simulink model "Control_Logic_a"  (R2018b)
settings: Solver=VariableStepAuto  StartTime=Start_time  StopTime=Stop_time  RelTol=1e-3
values from neighbouring files (symbols this model uses):
  Aset_N1 = 2    [Parameter_control.m]
  Aset_N10 = -10    [Parameter_control.m]
  Aset_N11 = 10    [Parameter_control.m]
  Aset_N12 = 20    [Parameter_control.m]
  Aset_N13 = 20    [Parameter_control.m]
  Aset_N2 = 30    [Parameter_control.m]
  Aset_N3 = 3    [Parameter_control.m]
  Aset_N4 = 5    [Parameter_control.m]
  Aset_N5 = 1    [Parameter_control.m]
  Aset_N6 = 0    [Parameter_control.m]
  Aset_N7 = 0.01    [Parameter_control.m]
  Aset_N8 = 2    [Parameter_control.m]
  Aset_N9 = 0.1    [Parameter_control.m]
  Dset_N1 = 1    [Parameter_control.m]
  Dset_N2 = 1    [Parameter_control.m]
  Ini_time = Start_time    (= 0)    [main.m]
  Sample_time = 0.1    [main.m]    (also in manual_env_for_test_slx.m; test_tool_initialize.m)
undefined symbols (not defined in the file or in its folder): DiscIntNeverNeededParam
(part 1 of 2)
settings Model: Creator=M156732  LastModifiedBy=M156732
settings ModelReferenceCC: ModelReferenceNumInstancesAllowed=Single

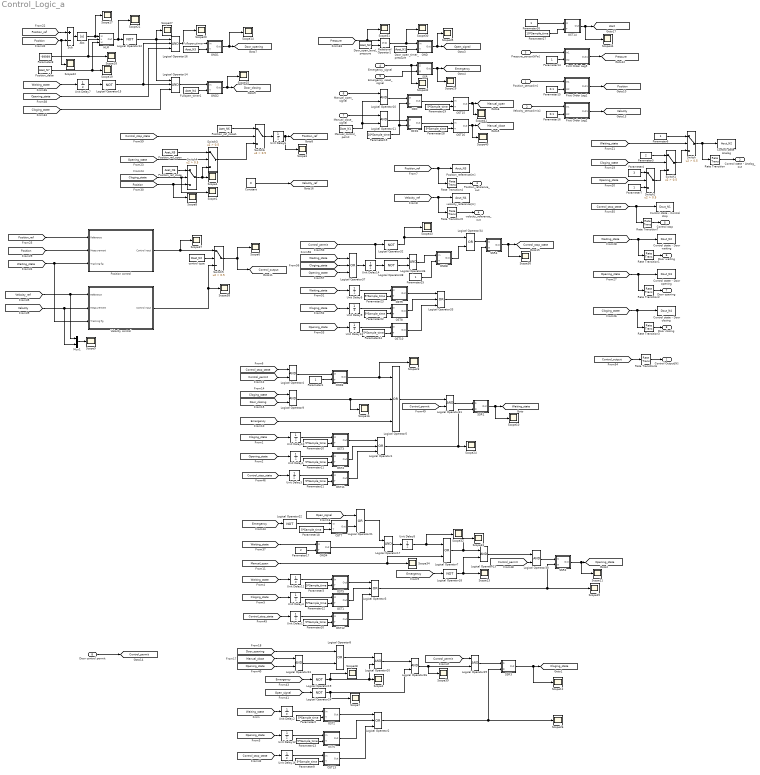
== system Control_Logic_a ==
  Position_sensor[m] : Inport  OutDataTypeStr=double  Unit=mm  SampleTime=Sample_time
  Velocity_sensor[m/s] : Inport  Port=2  OutDataTypeStr=double  Unit=mm  SampleTime=Sample_time
  Pressure_sensor[kPa] : Inport  Port=3  OutDataTypeStr=double  Unit=kPa  SampleTime=Sample_time
  Emergency_signal : Inport  Port=4  OutDataTypeStr=boolean  SampleTime=Sample_time
  Emergency_reset_signal : Inport  Port=5  OutDataTypeStr=boolean  SampleTime=Sample_time
  Manual_open_signal : Inport  Port=6  OutDataTypeStr=boolean  SampleTime=Sample_time
  Manual_close_signal : Inport  Port=7  OutDataTypeStr=boolean  SampleTime=Sample_time
  Door control permit : Inport  Port=8  OutDataTypeStr=boolean  SampleTime=Sample_time
  Abs : Abs
  Constant : Constant  Value=0
  Control state - Analog : ToWorkspace  VariableName=Aout_N2  SampleTime=Sample_time
  Control state - Control stop : ToWorkspace  VariableName=Dout_N1  SampleTime=Sample_time
  Control state - Door closing : ToWorkspace  VariableName=Dout_N4  SampleTime=Sample_time
  Control state - Door opening : ToWorkspace  VariableName=Dout_N3  SampleTime=Sample_time
  Control state - Door waiting : ToWorkspace  VariableName=Dout_N2  SampleTime=Sample_time
  Door_open_level_pressure : Constant  Value=Aset_N2  OutDataTypeStr=double  SampleTime=Sample_time
  Door_open_timer_pressure : Constant  Value=Aset_N1  OutDataTypeStr=double  SampleTime=Sample_time
  First Order Lag1 : Subsystem
  First Order Lag2 : Subsystem
  First Order Lag5 : Subsystem
  Fullopen_timer : Constant  Value=Aset_N3  OutDataTypeStr=double  SampleTime=Sample_time
  Fullopen_timer1 : Constant  Value=Aset_N4  OutDataTypeStr=double  SampleTime=Sample_time
  HLM : Subsystem
  Logical Operator{1..3,5,33,37} (6 alike) : Logic  Operator=OR  Inputs=3  AllPortsSameDT=off  OutDataTypeStr=boolean
  Logical Operator{4,9..11,13,17,20,23,26,29..31,36} (13 alike) : Logic  AllPortsSameDT=off  OutDataTypeStr=boolean
  Logical Operator{12,15,18..19,22,24,32,38} (8 alike) : Logic  Operator=NOT  AllPortsSameDT=off  OutDataTypeStr=boolean
  Logical Operator14 : Logic  Inputs=3  AllPortsSameDT=off  OutDataTypeStr=boolean
  Logical Operator16 : Logic  Inputs=3  AllPortsSameDT=off  OutDataTypeStr=boolean
  Logical Operator{7..8,21,34} (4 alike) : Logic  Operator=OR  AllPortsSameDT=off  OutDataTypeStr=boolean
  Manual_control_pemit : Constant  Value=Dset_N1  OutDataTypeStr=double  SampleTime=Sample_time
  Mux1 : Mux  Inputs=2
  OFD : Subsystem
  OFD1 : Subsystem
  OND : Subsystem
  OND1 : Subsystem
  OND2 : Subsystem
  OND3 : Subsystem
  OND4 : Subsystem
  OND8 : Subsystem
  OST1 : Subsystem
  OST10 : Subsystem
  OST11 : Subsystem
  OST12 : Subsystem
  OST13 : Subsystem
  OST14 : Subsystem
  OST15 : Subsystem
  OST16 : Subsystem
  OST2 : Subsystem
  OST3 : Subsystem
  OST4 : Subsystem
  OST5 : Subsystem
  OST6 : Subsystem
  OST7 : Subsystem
  OST8 : Subsystem
  OST9 : Subsystem
  Parameter{1,6..7,25} (4 alike) : Constant  OutDataTypeStr=int32  SampleTime=Sample_time
  Parameter{2..3,9..13,18,20..24,28..29} (15 alike) : Constant  Value=5*Sample_time  OutDataTypeStr=double  SampleTime=Sample_time
  Parameter14 : Constant  OutDataTypeStr=double  SampleTime=Sample_time
  Parameter15 : Constant  Value=0.1  OutDataTypeStr=double  SampleTime=Sample_time
  Parameter16 : Constant  Value=0.1  OutDataTypeStr=double  SampleTime=Sample_time
  Parameter17 : Constant  Value=2  OutDataTypeStr=int32  SampleTime=Sample_time
  Parameter19 : Constant  Value=10*Sample_time  OutDataTypeStr=double  SampleTime=Sample_time
  Parameter26 : Constant  OutDataTypeStr=boolean  SampleTime=Sample_time
  Parameter27 : Constant  Value=10*Sample_time  OutDataTypeStr=double  SampleTime=Sample_time
  Parameter4 : Constant  Value=3  OutDataTypeStr=int32  SampleTime=Sample_time
  Parameter5 : Constant  Value=2  OutDataTypeStr=int32  SampleTime=Sample_time
  Parameter8 : Constant  Value=-99999  OutDataTypeStr=double  SampleTime=Sample_time
  Position control : Subsystem
  Position_delta : Constant  Value=Aset_N7  OutDataTypeStr=double  SampleTime=Sample_time
  Position_ref_close : Constant  Value=Aset_N6  OutDataTypeStr=double  SampleTime=Sample_time
  Position_ref_close1 : Constant  Value=Aset_N6  OutDataTypeStr=double  SampleTime=Sample_time
  Position_ref_open : Constant  Value=Aset_N5  OutDataTypeStr=double  SampleTime=Sample_time
  Position_reference[m] : ToWorkspace  VariableName=Aout_N3  SampleTime=Sample_time
  Rate Transition{,1..7} (8 alike) : RateTransition  OutPortSampleTime=Sample_time
  Relational Operator1 : RelationalOperator  OutDataTypeStr=boolean  RndMeth=Nearest
  SSR : Subsystem
  SSR1 : Subsystem
  SSR2 : Subsystem
  SSR3 : Subsystem
  SSR4 : Subsystem
  Scope{1..4,6..44} (43 alike) : Scope
  Sub : Sum  Inputs=+-  OutDataTypeStr=double
  Switch : Switch  Criteria=u2 > Threshold  Threshold=0.5  OutDataTypeStr=int32
  Switch1 : Switch  Criteria=u2 > Threshold  Threshold=0.5  OutDataTypeStr=int32
  Switch2 : Switch  Criteria=u2 > Threshold  Threshold=0.5  OutDataTypeStr=int32
  Switch{3..6} (4 alike) : Switch  Criteria=u2 > Threshold  Threshold=0.5  OutDataTypeStr=double
  Unit Delay{1..13,15..16} (15 alike) : UnitDelay  SampleTime=Sample_time
  Unit Delay14 : UnitDelay  InitialCondition=1  SampleTime=Sample_time
  Velocity control : Subsystem
  control type : Constant  Value=Dset_N2  OutDataTypeStr=double  SampleTime=Sample_time
  velocity_reference[m] : ToWorkspace  VariableName=Aout_N4  SampleTime=Sample_time
  Control Output[N] : Outport  OutDataTypeStr=double  Unit=N  SampleTime=Sample_time  LockScale=on
  Control state - Analog_out : Outport  Port=2  SampleTime=Sample_time
  Position_reference_out : Outport  Port=3  SampleTime=Sample_time
  velocity_reference_out : Outport  Port=4  SampleTime=Sample_time
  Control stop : Outport  Port=5  SampleTime=Sample_time
  Door waiting : Outport  Port=6  SampleTime=Sample_time
  Door opening : Outport  Port=7  SampleTime=Sample_time
  Door closing : Outport  Port=8  SampleTime=Sample_time
  tag scope: Cloging_state=global, Control_output=global, Control_permit=global, Control_stop_state=global, Door_closing=global, Door_opening=global, Emergency=global, Manual_close=global, Manual_open=global, Open_signal=global, Opening_state=global, Position=global, Position_ref=global, Pressure=global, Velocity=global, Velocity_ref=global, Waiting_state=global, start=global
  wires:
  SSR1/1(Out) -> Scope10/1, [Waiting_state]
  SSR3/1(Out) -> Scope12/1, [Cloging_state]
  SSR2/1(Out) -> Scope11/1, [Opening_state]
  Logical Operator9/1 -> Scope16/1, Logical Operator5/2
  [Emergency] -> Logical Operator5/3
  [Door_closing] -> Logical Operator9/2
  [Cloging_state] -> Logical Operator9/1
  [Manual_open] -> Scope34/1, Logical Operator7/2
  Logical Operator7/1 -> Logical Operator13/1, Scope33/1
  [Door_opening] -> Logical Operator8/1
  Door_open_timer_pressure/1 -> OND/2(T)
  Door_open_level_pressure/1 -> Relational Operator1/2
  Relational Operator1/1 -> Scope30/1, OND/1(In)
  OND/1(Out) -> Scope35/1, [Open_signal]
  SSR/1(Out) -> Scope29/1, [Emergency]
  Emergency_reset_signal/1 -> SSR/2(R)
  Switch1/1 -> Switch/3
  Switch2/1 -> Switch1/3
  Parameter4/1 -> Switch2/1
  Parameter5/1 -> Switch1/1
  Parameter6/1 -> Switch/1
  Parameter7/1 -> Switch2/3
  Switch/1 -> Rate Transition/1, Control state - Analog/1
  Manual_control_pemit/1 -> Logical Operator10/2, Logical Operator11/2
  [Position_ref] -> Sub/1
  Sub/1 -> Abs/1
  Position_delta/1 -> Scope19/1, HLM/3(H)
  Parameter8/1 -> Scope18/1, HLM/2(L)
  HLM/1(Out) -> Scope21/1, Logical Operator12/1
  Fullopen_timer/1 -> OND1/2(T)
  [Opening_state] -> Switch3/2
  Switch4/1 -> Scope4/1, Switch3/3
  [Cloging_state] -> Scope1/1, Switch4/2
  Position_ref_open/1 -> Switch3/1
  Position_ref_close/1 -> Switch4/1
  [Position] -> Scope8/1, Switch4/3
  Fullopen_timer1/1 -> OND2/2(T)
  [Waiting_state] -> Rate Transition1/1, Control state - Door waiting/1
  [Opening_state] -> Rate Transition2/1, Control state - Door opening/1
  [Cloging_state] -> Rate Transition3/1, Control state - Door closing/1
  [Position] -> Scope22/1, Sub/2
  Unit Delay6/1 -> Scope3/1, [Position_ref]
  [Pressure] -> Scope31/1, Relational Operator1/1
  Parameter1/1 -> OND3/2(T)
  Logical Operator4/1 -> OND3/1(In)
  OND3/1(Out) -> Scope23/1, Logical Operator5/1
  Abs/1 -> Scope17/1, HLM/1(In)
  OND1/1(Out) -> Scope14/1, [Door_opening]
  OND2/1(Out) -> Scope15/1, [Door_closing]
  [Waiting_state] -> Unit Delay7/1
  Logical Operator12/1 -> Logical Operator16/1, Scope27/1, Logical Operator14/1
  Logical Operator16/1 -> OND1/1(In), Scope20/1
  Logical Operator15/1 -> Logical Operator14/2, Logical Operator16/2
  Unit Delay7/1 -> Logical Operator15/1
  Logical Operator1/1 -> SSR1/2(R), Scope24/1
  Logical Operator17/1 -> Unit Delay8/1
  Unit Delay8/1 -> Scope32/1, Logical Operator7/1
  [Opening_state] -> Logical Operator16/3
  [Cloging_state] -> Logical Operator14/3
  Logical Operator14/1 -> OND2/1(In)
  [Opening_state] -> Unit Delay1/1
  [Cloging_state] -> Unit Delay10/1
  Parameter10/1 -> OST3/2(T)
  OST3/1(Out) -> Logical Operator1/1
  Unit Delay10/1 -> OST3/1(In)
  Unit Delay1/1 -> OST4/1(In)
  Parameter11/1 -> OST4/2(T)
  OST4/1(Out) -> Logical Operator1/2
  Parameter12/1 -> OST1/2(T)
  Logical Operator3/1 -> SSR2/2(R), Scope25/1
  OST1/1(Out) -> Logical Operator3/2
  Parameter3/1 -> OST5/2(T)
  [Waiting_state] -> Unit Delay11/1
  OST5/1(Out) -> Logical Operator3/1
  Unit Delay11/1 -> OST5/1(In)
  [Cloging_state] -> Unit Delay4/1
  Unit Delay4/1 -> OST1/1(In)
  [Waiting_state] -> Unit Delay2/1
  Parameter2/1 -> OST2/2(T)
  Logical Operator2/1 -> Scope26/1, SSR3/2(R)
  OST2/1(Out) -> Logical Operator2/1
  Parameter13/1 -> OST6/2(T)
  [Opening_state] -> Unit Delay12/1
  OST6/1(Out) -> Logical Operator2/2
  Unit Delay2/1 -> OST2/1(In)
  Unit Delay12/1 -> OST6/1(In)
  [Position_ref] -> Position control/1(Reference)
  [Position] -> Position control/2(Measurement)
  [Waiting_state] -> Velocity control/3(Tracking flg), Position control/3(Tracking flg)
  Position control/1(Control input) -> Scope37/1, Switch5/1
  Switch5/1 -> Scope6/1, [Control_output]
  Velocity control/1(Control input) -> Scope38/1, Switch5/3
  control type/1 -> Switch5/2
  [Velocity] -> Velocity control/2(Measurement), Mux1/2
  [Velocity_ref] -> Velocity control/1(Reference), Mux1/1
  Mux1/1 -> Scope9/1
  Pressure_sensor[kPa]/1 -> First Order Lag5/1(In1)
  First Order Lag5/1(Out1) -> [Pressure]
  First Order Lag1/1(Out1) -> [Position]
  Position_sensor[m]/1 -> First Order Lag1/1(In1)
  First Order Lag2/1(Out1) -> [Velocity]
  Velocity_sensor[m/s]/1 -> First Order Lag2/1(In1)
  Parameter14/1 -> First Order Lag5/2(In2)
  Parameter15/1 -> First Order Lag1/2(In2)
  Parameter16/1 -> First Order Lag2/2(In2)
  [Waiting_state] -> Switch/2
  [Cloging_state] -> Switch1/2
  [Opening_state] -> Switch2/2
  Rate Transition/1 -> Control state - Analog_out/1
  Rate Transition1/1 -> Door waiting/1
  Rate Transition2/1 -> Door opening/1
  Rate Transition3/1 -> Door closing/1
  Parameter17/1 -> OND4/2(T)
  [Waiting_state] -> OND4/1(In)
  OND4/1(Out) -> Logical Operator17/2
  [Position_ref] -> Rate Transition4/1, Position_reference[m]/1
  Rate Transition4/1 -> Position_reference_out/1
  Rate Transition5/1 -> velocity_reference_out/1
  [Velocity_ref] -> velocity_reference[m]/1, Rate Transition5/1
  [Emergency] -> Logical Operator18/1
  Logical Operator18/1 -> Scope13/1, Logical Operator13/2
  [Emergency] -> Logical Operator19/1
  Logical Operator8/1 -> Logical Operator20/1
  Logical Operator21/1 -> Logical Operator17/1
  [Open_signal] -> Logical Operator21/1
  [Emergency] -> Logical Operator22/1
  Parameter18/1 -> OST7/2(T)
  OST7/1(Out) -> Logical Operator21/2
  Logical Operator22/1 -> OST7/1(In)
  Manual_open_signal/1 -> Logical Operator10/1
  Manual_close_signal/1 -> Logical Operator11/1
  Logical Operator11/1 -> OFD1/1(In)
  Logical Operator10/1 -> OFD/1(In)
  Parameter19/1 -> OFD1/2(T), OFD/2(T)
  [Manual_close] -> Logical Operator23/1
  Logical Operator23/1 -> Logical Operator8/2
  [Opening_state] -> Logical Operator23/2
  [Open_signal] -> Logical Operator24/1
  Logical Operator24/1 -> Scope7/1, Logical Operator26/2
  Logical Operator19/1 -> Logical Operator20/2, Scope2/1, Scope28/1
  Emergency_signal/1 -> Scope42/1, SSR/1(S)
  Logical Operator20/1 -> Logical Operator26/1
  OST13/1(Out) -> Logical Operator2/3
  Door control permit/1 -> [Control_permit]
  OST12/1(Out) -> Logical Operator3/3
  OST11/1(Out) -> Logical Operator1/3
  Logical Operator29/1 -> SSR3/1(S)
  Logical Operator26/1 -> Scope39/1, Logical Operator29/2
  [Control_permit] -> Logical Operator29/1
  Logical Operator13/1 -> Logical Operator30/1
  Logical Operator30/1 -> SSR2/1(S)
  [Control_permit] -> Logical Operator30/2
  [Control_permit] -> Logical Operator31/2
  Logical Operator5/1 -> Logical Operator31/1
  Logical Operator31/1 -> SSR1/1(S)
  SSR4/1(Out) -> Scope36/1, [Control_stop_state]
  [Control_permit] -> Logical Operator36/1, Logical Operator32/1
  OST10/1(Out) -> Logical Operator33/3
  Unit Delay9/1 -> OST8/1(In)
  [Cloging_state] -> Unit Delay9/1
  Unit Delay5/1 -> OST9/1(In)
  OST9/1(Out) -> Logical Operator33/1
  [Waiting_state] -> Unit Delay5/1
  Parameter23/1 -> OST9/2(T)
  OST8/1(Out) -> Logical Operator33/2
  Parameter22/1 -> OST8/2(T)
  Parameter24/1 -> OST10/2(T)
  Unit Delay13/1 -> OST10/1(In)
  [Opening_state] -> Unit Delay13/1
  Logical Operator33/1 -> SSR4/2(R)
  Rate Transition6/1 -> Control Output[N]/1
  [Control_output] -> Rate Transition6/1
  Rate Transition7/1 -> Control stop/1
  [Control_stop_state] -> Control state - Control stop/1, Rate Transition7/1
  Constant/1 -> [Velocity_ref]
  Logical Operator32/1 -> Logical Operator34/1, Scope43/1
  Logical Operator34/1 -> SSR4/1(S)
  [Cloging_state] -> Logical Operator37/2
  Unit Delay14/1 -> Logical Operator38/1
  [Waiting_state] -> Logical Operator37/1
  Logical Operator37/1 -> Unit Delay14/1
  [Opening_state] -> Logical Operator37/3
  Parameter25/1 -> OND8/2(T)
  [Control_stop_state] -> Logical Operator4/1
  [Control_permit] -> Logical Operator4/2
  Parameter26/1 -> OST14/1(In)
  OST14/1(Out) -> Scope44/1, [start]
  Parameter27/1 -> OST14/2(T)
  Logical Operator36/1 -> OND8/1(In)
  Logical Operator38/1 -> Logical Operator36/2
  Parameter21/1 -> OST11/2(T)
  Unit Delay3/1 -> OST11/1(In)
  [Control_stop_state] -> Unit Delay3/1
  [Control_stop_state] -> Unit Delay15/1
  Unit Delay15/1 -> OST12/1(In)
  Parameter20/1 -> OST12/2(T)
  Parameter9/1 -> OST13/2(T)
  Unit Delay16/1 -> OST13/1(In)
  [Control_stop_state] -> Unit Delay16/1
  Switch3/1 -> Switch6/3
  Switch6/1 -> Unit Delay6/1
  [Control_stop_state] -> Switch6/2
  Position_ref_close1/1 -> Switch6/1
  OFD/1(Out) -> OST15/1(In)
  OFD1/1(Out) -> OST16/1(In)
  Parameter28/1 -> OST16/2(T)
  Parameter29/1 -> OST15/2(T)
  OST16/1(Out) -> Scope40/1, [Manual_close]
  OST15/1(Out) -> Scope41/1, [Manual_open]
  OND8/1(Out) -> Logical Operator34/2

== system Control_Logic_a/First Order Lag1 ==
  In1 : Inport
  In2 : Inport  Port=2
  Discrete-Time Integrator : DiscreteIntegrator  InitialConditionSource=external  SampleTime=Sample_time  ICPrevOutput=DiscIntNeverNeededParam  ICPrevScaledInput=DiscIntNeverNeededParam
  Product : Product  Inputs=*/  SaturateOnIntegerOverflow=on  OutDataTypeStr=Inherit: Same as first input
  Sum : Sum  Inputs=|+-  SaturateOnIntegerOverflow=on
  Out1 : Outport
  wires:
  In1/1 -> Sum/1, Discrete-Time Integrator/2
  Discrete-Time Integrator/1 -> Out1/1, Sum/2
  Product/1 -> Discrete-Time Integrator/1
  Sum/1 -> Product/1
  In2/1 -> Product/2

== system Control_Logic_a/First Order Lag2 ==
  In1 : Inport
  In2 : Inport  Port=2
  Discrete-Time Integrator : DiscreteIntegrator  InitialConditionSource=external  SampleTime=Sample_time  ICPrevOutput=DiscIntNeverNeededParam  ICPrevScaledInput=DiscIntNeverNeededParam
  Product : Product  Inputs=*/  SaturateOnIntegerOverflow=on  OutDataTypeStr=Inherit: Same as first input
  Sum : Sum  Inputs=|+-  SaturateOnIntegerOverflow=on
  Out1 : Outport
  wires:
  In2/1 -> Product/2
  Sum/1 -> Product/1
  Product/1 -> Discrete-Time Integrator/1
  Discrete-Time Integrator/1 -> Sum/2, Out1/1
  In1/1 -> Discrete-Time Integrator/2, Sum/1

== system Control_Logic_a/First Order Lag5 ==
  In1 : Inport
  In2 : Inport  Port=2
  Discrete-Time Integrator : DiscreteIntegrator  InitialConditionSource=external  SampleTime=Sample_time  ICPrevOutput=DiscIntNeverNeededParam  ICPrevScaledInput=DiscIntNeverNeededParam
  Product : Product  Inputs=*/  SaturateOnIntegerOverflow=on  OutDataTypeStr=Inherit: Same as first input
  Sum : Sum  Inputs=|+-  SaturateOnIntegerOverflow=on
  Out1 : Outport
  wires:
  In2/1 -> Product/2
  Sum/1 -> Product/1
  Product/1 -> Discrete-Time Integrator/1
  Discrete-Time Integrator/1 -> Sum/2, Out1/1
  In1/1 -> Discrete-Time Integrator/2, Sum/1

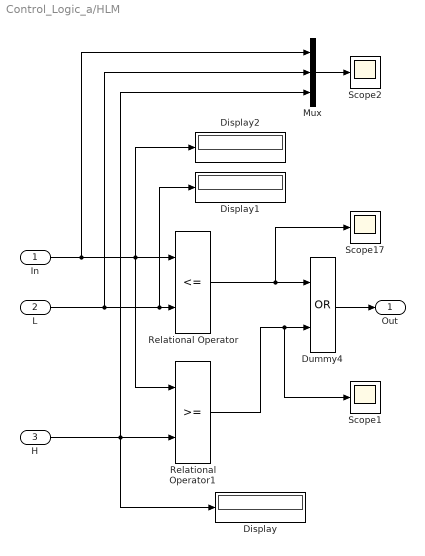
== system Control_Logic_a/HLM ==
  In : Inport
  L : Inport  Port=2
  H : Inport  Port=3
  Display : Display
  Display1 : Display
  Display2 : Display
  Dummy4 : Logic  Operator=OR  AllPortsSameDT=off  OutDataTypeStr=boolean
  Mux : Mux  Inputs=3
  Relational Operator : RelationalOperator  Operator=<=  OutDataTypeStr=boolean  RndMeth=Nearest
  Relational Operator1 : RelationalOperator  OutDataTypeStr=boolean  RndMeth=Nearest
  Scope1 : Scope
  Scope17 : Scope
  Scope2 : Scope
  Out : Outport
  wires:
  Dummy4/1 -> Out/1
  Relational Operator1/1 -> Scope1/1, Dummy4/2
  Relational Operator/1 -> Scope17/1, Dummy4/1
  H/1 -> Display/1, Mux/3, Relational Operator1/2
  In/1 -> Mux/1, Display2/1, Relational Operator1/1, Relational Operator/1
  L/1 -> Mux/2, Display1/1, Relational Operator/2
  Mux/1 -> Scope2/1

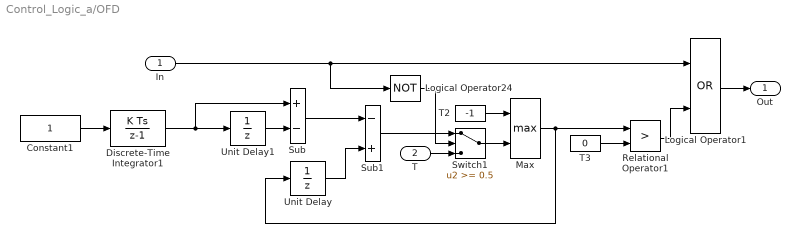
== system Control_Logic_a/OFD ==
  In : Inport
  T : Inport  Port=2  SampleTime=Sample_time
  Constant1 : Constant  SampleTime=Sample_time
  Discrete-Time Integrator1 : DiscreteIntegrator  SampleTime=Sample_time  LimitOutput=on  LowerSaturationLimit=0  ICPrevOutput=DiscIntNeverNeededParam  ICPrevScaledInput=DiscIntNeverNeededParam
  Logical Operator1 : Logic  Operator=OR  AllPortsSameDT=off  OutDataTypeStr=boolean
  Logical Operator24 : Logic  Operator=NOT  AllPortsSameDT=off  OutDataTypeStr=boolean
  Max : MinMax  Function=max  Inputs=2  OutDataTypeStr=double
  Relational Operator1 : RelationalOperator  Operator=>  OutDataTypeStr=boolean  RndMeth=Nearest
  Sub : Sum  Inputs=+-  OutDataTypeStr=double
  Sub1 : Sum  Inputs=-+
  Switch1 : Switch  Threshold=0.5  OutDataTypeStr=double
  T2 : Constant  Value=-1
  T3 : Constant  Value=0
  Unit Delay : UnitDelay  SampleTime=Sample_time
  Unit Delay1 : UnitDelay  InitialCondition=Ini_time  SampleTime=Sample_time
  Out : Outport
  wires:
  In/1 -> Logical Operator1/1, Logical Operator24/1
  Logical Operator1/1 -> Out/1
  Relational Operator1/1 -> Logical Operator1/2
  Switch1/1 -> Max/2
  T/1 -> Switch1/3
  Unit Delay/1 -> Sub1/2
  Sub/1 -> Sub1/1
  Unit Delay1/1 -> Sub/2
  Sub1/1 -> Switch1/1
  Discrete-Time Integrator1/1 -> Unit Delay1/1, Sub/1
  Max/1 -> Relational Operator1/1, Unit Delay/1
  T3/1 -> Relational Operator1/2
  T2/1 -> Max/1
  Logical Operator24/1 -> Switch1/2
  Constant1/1 -> Discrete-Time Integrator1/1

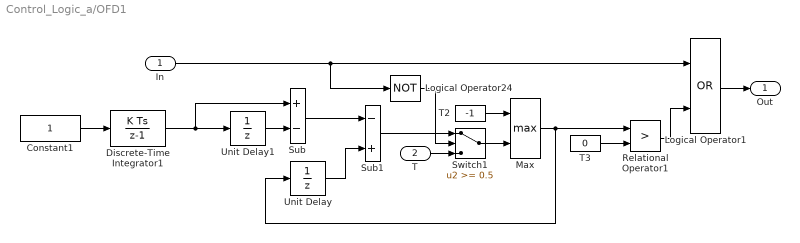
== system Control_Logic_a/OFD1 ==
  In : Inport
  T : Inport  Port=2  SampleTime=Sample_time
  Constant1 : Constant  SampleTime=Sample_time
  Discrete-Time Integrator1 : DiscreteIntegrator  SampleTime=Sample_time  LimitOutput=on  LowerSaturationLimit=0  ICPrevOutput=DiscIntNeverNeededParam  ICPrevScaledInput=DiscIntNeverNeededParam
  Logical Operator1 : Logic  Operator=OR  AllPortsSameDT=off  OutDataTypeStr=boolean
  Logical Operator24 : Logic  Operator=NOT  AllPortsSameDT=off  OutDataTypeStr=boolean
  Max : MinMax  Function=max  Inputs=2  OutDataTypeStr=double
  Relational Operator1 : RelationalOperator  Operator=>  OutDataTypeStr=boolean  RndMeth=Nearest
  Sub : Sum  Inputs=+-  OutDataTypeStr=double
  Sub1 : Sum  Inputs=-+
  Switch1 : Switch  Threshold=0.5  OutDataTypeStr=double
  T2 : Constant  Value=-1
  T3 : Constant  Value=0
  Unit Delay : UnitDelay  SampleTime=Sample_time
  Unit Delay1 : UnitDelay  InitialCondition=Ini_time  SampleTime=Sample_time
  Out : Outport
  wires:
  Constant1/1 -> Discrete-Time Integrator1/1
  Logical Operator24/1 -> Switch1/2
  T2/1 -> Max/1
  T3/1 -> Relational Operator1/2
  Max/1 -> Unit Delay/1, Relational Operator1/1
  Discrete-Time Integrator1/1 -> Sub/1, Unit Delay1/1
  Sub1/1 -> Switch1/1
  Unit Delay1/1 -> Sub/2
  Sub/1 -> Sub1/1
  Unit Delay/1 -> Sub1/2
  T/1 -> Switch1/3
  Switch1/1 -> Max/2
  Relational Operator1/1 -> Logical Operator1/2
  Logical Operator1/1 -> Out/1
  In/1 -> Logical Operator24/1, Logical Operator1/1

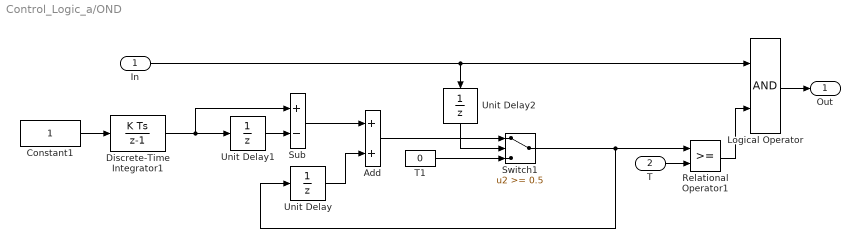
== system Control_Logic_a/OND ==
  In : Inport
  T : Inport  Port=2
  Add : Sum  OutDataTypeStr=double
  Constant1 : Constant  SampleTime=Sample_time
  Discrete-Time Integrator1 : DiscreteIntegrator  SampleTime=Sample_time  LimitOutput=on  LowerSaturationLimit=0  ICPrevOutput=DiscIntNeverNeededParam  ICPrevScaledInput=DiscIntNeverNeededParam
  Logical Operator : Logic  AllPortsSameDT=off  OutDataTypeStr=boolean
  Relational Operator1 : RelationalOperator  OutDataTypeStr=boolean  RndMeth=Nearest
  Sub : Sum  Inputs=+-  AccumDataTypeStr=double
  Switch1 : Switch  Threshold=0.5  OutDataTypeStr=double
  T1 : Constant  Value=0  OutDataTypeStr=double
  Unit Delay : UnitDelay  SampleTime=Sample_time
  Unit Delay1 : UnitDelay  InitialCondition=Ini_time  SampleTime=Sample_time
  Unit Delay2 : UnitDelay  SampleTime=Sample_time
  Out : Outport
  wires:
  Unit Delay2/1 -> Switch1/2
  Discrete-Time Integrator1/1 -> Sub/1, Unit Delay1/1
  Add/1 -> Switch1/1
  Unit Delay1/1 -> Sub/2
  Sub/1 -> Add/1
  Unit Delay/1 -> Add/2
  T1/1 -> Switch1/3
  Switch1/1 -> Relational Operator1/1, Unit Delay/1
  T/1 -> Relational Operator1/2
  Relational Operator1/1 -> Logical Operator/2
  Logical Operator/1 -> Out/1
  In/1 -> Unit Delay2/1, Logical Operator/1
  Constant1/1 -> Discrete-Time Integrator1/1

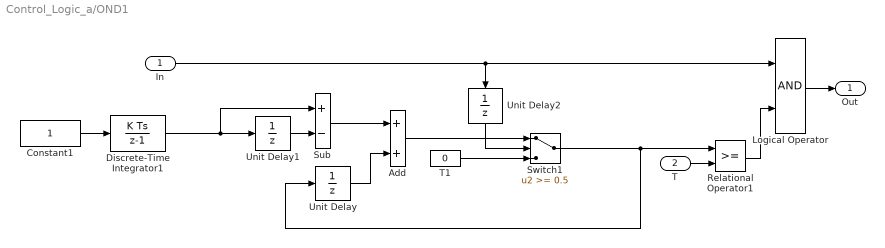
== system Control_Logic_a/OND1 ==
  In : Inport
  T : Inport  Port=2
  Add : Sum  OutDataTypeStr=double
  Constant1 : Constant  SampleTime=Sample_time
  Discrete-Time Integrator1 : DiscreteIntegrator  SampleTime=Sample_time  LimitOutput=on  LowerSaturationLimit=0  ICPrevOutput=DiscIntNeverNeededParam  ICPrevScaledInput=DiscIntNeverNeededParam
  Logical Operator : Logic  AllPortsSameDT=off  OutDataTypeStr=boolean
  Relational Operator1 : RelationalOperator  OutDataTypeStr=boolean  RndMeth=Nearest
  Sub : Sum  Inputs=+-  AccumDataTypeStr=double
  Switch1 : Switch  Threshold=0.5  OutDataTypeStr=double
  T1 : Constant  Value=0  OutDataTypeStr=double
  Unit Delay : UnitDelay  SampleTime=Sample_time
  Unit Delay1 : UnitDelay  InitialCondition=Ini_time  SampleTime=Sample_time
  Unit Delay2 : UnitDelay  SampleTime=Sample_time
  Out : Outport
  wires:
  In/1 -> Logical Operator/1, Unit Delay2/1
  Logical Operator/1 -> Out/1
  Relational Operator1/1 -> Logical Operator/2
  T/1 -> Relational Operator1/2
  Switch1/1 -> Unit Delay/1, Relational Operator1/1
  T1/1 -> Switch1/3
  Unit Delay/1 -> Add/2
  Sub/1 -> Add/1
  Unit Delay1/1 -> Sub/2
  Add/1 -> Switch1/1
  Discrete-Time Integrator1/1 -> Unit Delay1/1, Sub/1
  Unit Delay2/1 -> Switch1/2
  Constant1/1 -> Discrete-Time Integrator1/1

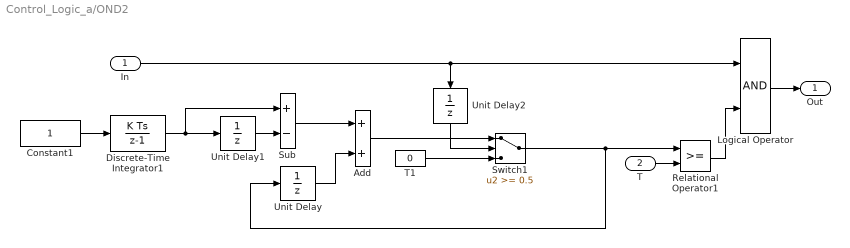
== system Control_Logic_a/OND2 ==
  In : Inport
  T : Inport  Port=2
  Add : Sum  OutDataTypeStr=double
  Constant1 : Constant  SampleTime=Sample_time
  Discrete-Time Integrator1 : DiscreteIntegrator  SampleTime=Sample_time  LimitOutput=on  LowerSaturationLimit=0  ICPrevOutput=DiscIntNeverNeededParam  ICPrevScaledInput=DiscIntNeverNeededParam
  Logical Operator : Logic  AllPortsSameDT=off  OutDataTypeStr=boolean
  Relational Operator1 : RelationalOperator  OutDataTypeStr=boolean  RndMeth=Nearest
  Sub : Sum  Inputs=+-  AccumDataTypeStr=double
  Switch1 : Switch  Threshold=0.5  OutDataTypeStr=double
  T1 : Constant  Value=0  OutDataTypeStr=double
  Unit Delay : UnitDelay  SampleTime=Sample_time
  Unit Delay1 : UnitDelay  InitialCondition=Ini_time  SampleTime=Sample_time
  Unit Delay2 : UnitDelay  SampleTime=Sample_time
  Out : Outport
  wires:
  Unit Delay2/1 -> Switch1/2
  Discrete-Time Integrator1/1 -> Sub/1, Unit Delay1/1
  Add/1 -> Switch1/1
  Unit Delay1/1 -> Sub/2
  Sub/1 -> Add/1
  Unit Delay/1 -> Add/2
  T1/1 -> Switch1/3
  Switch1/1 -> Relational Operator1/1, Unit Delay/1
  T/1 -> Relational Operator1/2
  Relational Operator1/1 -> Logical Operator/2
  Logical Operator/1 -> Out/1
  In/1 -> Unit Delay2/1, Logical Operator/1
  Constant1/1 -> Discrete-Time Integrator1/1

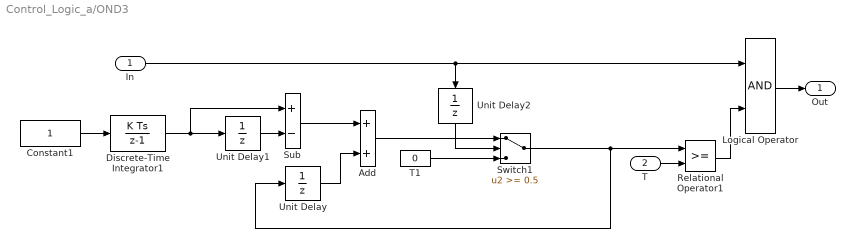
== system Control_Logic_a/OND3 ==
  In : Inport
  T : Inport  Port=2
  Add : Sum  OutDataTypeStr=double
  Constant1 : Constant  SampleTime=Sample_time
  Discrete-Time Integrator1 : DiscreteIntegrator  SampleTime=Sample_time  LimitOutput=on  LowerSaturationLimit=0  ICPrevOutput=DiscIntNeverNeededParam  ICPrevScaledInput=DiscIntNeverNeededParam
  Logical Operator : Logic  AllPortsSameDT=off  OutDataTypeStr=boolean
  Relational Operator1 : RelationalOperator  OutDataTypeStr=boolean  RndMeth=Nearest
  Sub : Sum  Inputs=+-  AccumDataTypeStr=double
  Switch1 : Switch  Threshold=0.5  OutDataTypeStr=double
  T1 : Constant  Value=0  OutDataTypeStr=double
  Unit Delay : UnitDelay  SampleTime=Sample_time
  Unit Delay1 : UnitDelay  InitialCondition=Ini_time  SampleTime=Sample_time
  Unit Delay2 : UnitDelay  SampleTime=Sample_time
  Out : Outport
  wires:
  In/1 -> Logical Operator/1, Unit Delay2/1
  Logical Operator/1 -> Out/1
  Relational Operator1/1 -> Logical Operator/2
  T/1 -> Relational Operator1/2
  Switch1/1 -> Unit Delay/1, Relational Operator1/1
  T1/1 -> Switch1/3
  Unit Delay/1 -> Add/2
  Sub/1 -> Add/1
  Unit Delay1/1 -> Sub/2
  Add/1 -> Switch1/1
  Discrete-Time Integrator1/1 -> Unit Delay1/1, Sub/1
  Unit Delay2/1 -> Switch1/2
  Constant1/1 -> Discrete-Time Integrator1/1

== system Control_Logic_a/OND4 ==
  In : Inport
  T : Inport  Port=2
  Add : Sum  OutDataTypeStr=double
  Clock : Clock
  Logical Operator : Logic  AllPortsSameDT=off  OutDataTypeStr=boolean
  Relational Operator1 : RelationalOperator  OutDataTypeStr=boolean  RndMeth=Nearest
  Sub : Sum  Inputs=+-  AccumDataTypeStr=double
  Switch1 : Switch  Threshold=0.5  OutDataTypeStr=double
  T1 : Constant  Value=0  OutDataTypeStr=double
  Unit Delay : UnitDelay  SampleTime=Sample_time
  Unit Delay1 : UnitDelay  InitialCondition=Ini_time  SampleTime=Sample_time
  Unit Delay2 : UnitDelay  SampleTime=Sample_time
  Out : Outport
  wires:
  In/1 -> Logical Operator/1, Unit Delay2/1
  Logical Operator/1 -> Out/1
  Relational Operator1/1 -> Logical Operator/2
  T/1 -> Relational Operator1/2
  Switch1/1 -> Unit Delay/1, Relational Operator1/1
  T1/1 -> Switch1/3
  Unit Delay/1 -> Add/2
  Sub/1 -> Add/1
  Unit Delay1/1 -> Sub/2
  Add/1 -> Switch1/1
  Clock/1 -> Unit Delay1/1, Sub/1
  Unit Delay2/1 -> Switch1/2

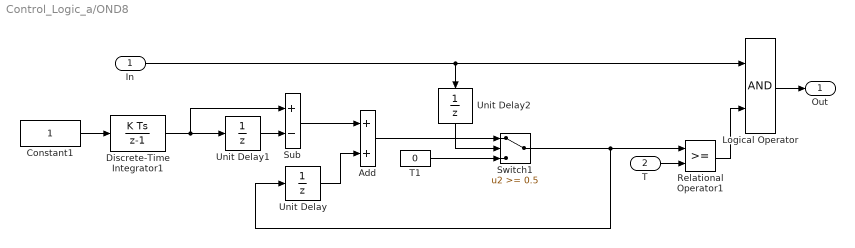
== system Control_Logic_a/OND8 ==
  In : Inport
  T : Inport  Port=2
  Add : Sum  OutDataTypeStr=double
  Constant1 : Constant  SampleTime=Sample_time
  Discrete-Time Integrator1 : DiscreteIntegrator  SampleTime=Sample_time  LimitOutput=on  LowerSaturationLimit=0  ICPrevOutput=DiscIntNeverNeededParam  ICPrevScaledInput=DiscIntNeverNeededParam
  Logical Operator : Logic  AllPortsSameDT=off  OutDataTypeStr=boolean
  Relational Operator1 : RelationalOperator  OutDataTypeStr=boolean  RndMeth=Nearest
  Sub : Sum  Inputs=+-  AccumDataTypeStr=double
  Switch1 : Switch  Threshold=0.5  OutDataTypeStr=double
  T1 : Constant  Value=0  OutDataTypeStr=double
  Unit Delay : UnitDelay  SampleTime=Sample_time
  Unit Delay1 : UnitDelay  InitialCondition=Ini_time  SampleTime=Sample_time
  Unit Delay2 : UnitDelay  SampleTime=Sample_time
  Out : Outport
  wires:
  Constant1/1 -> Discrete-Time Integrator1/1
  Unit Delay2/1 -> Switch1/2
  Discrete-Time Integrator1/1 -> Sub/1, Unit Delay1/1
  Add/1 -> Switch1/1
  Unit Delay1/1 -> Sub/2
  Sub/1 -> Add/1
  Unit Delay/1 -> Add/2
  T1/1 -> Switch1/3
  Switch1/1 -> Relational Operator1/1, Unit Delay/1
  T/1 -> Relational Operator1/2
  Relational Operator1/1 -> Logical Operator/2
  Logical Operator/1 -> Out/1
  In/1 -> Unit Delay2/1, Logical Operator/1

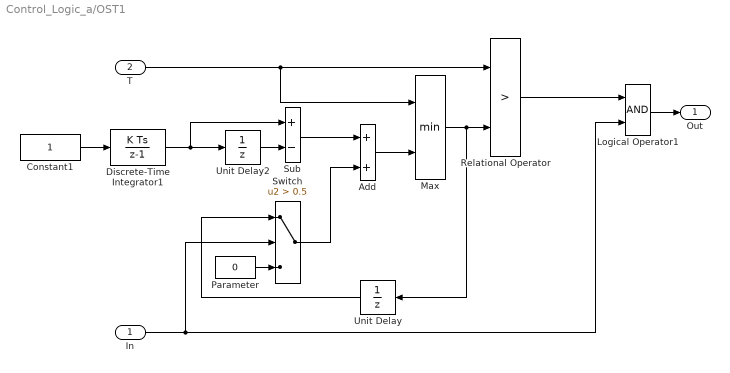
== system Control_Logic_a/OST1 ==
  In : Inport  OutDataTypeStr=boolean  SampleTime=Sample_time
  T : Inport  Port=2  OutDataTypeStr=double  SampleTime=Sample_time
  Add : Sum  OutDataTypeStr=double
  Constant1 : Constant  SampleTime=Sample_time
  Discrete-Time Integrator1 : DiscreteIntegrator  SampleTime=Sample_time  LimitOutput=on  LowerSaturationLimit=0  ICPrevOutput=DiscIntNeverNeededParam  ICPrevScaledInput=DiscIntNeverNeededParam
  Logical Operator1 : Logic  AllPortsSameDT=off  OutDataTypeStr=boolean
  Max : MinMax  Inputs=2  OutDataTypeStr=double
  Parameter : Constant  Value=0  OutDataTypeStr=double  SampleTime=Sample_time
  Relational Operator : RelationalOperator  Operator=>  OutDataTypeStr=boolean  RndMeth=Nearest
  Sub : Sum  Inputs=+-  AccumDataTypeStr=single  OutDataTypeStr=double
  Switch : Switch  Criteria=u2 > Threshold  Threshold=0.5  OutDataTypeStr=double
  Unit Delay : UnitDelay  SampleTime=Sample_time
  Unit Delay2 : UnitDelay  InitialCondition=Ini_time  SampleTime=Sample_time
  Out : Outport  OutDataTypeStr=boolean  SampleTime=Sample_time
  wires:
  In/1 -> Switch/2, Logical Operator1/2
  Discrete-Time Integrator1/1 -> Unit Delay2/1, Sub/1
  Unit Delay2/1 -> Sub/2
  Sub/1 -> Add/1
  Logical Operator1/1 -> Out/1
  Relational Operator/1 -> Logical Operator1/1
  Switch/1 -> Add/2
  Unit Delay/1 -> Switch/1
  Parameter/1 -> Switch/3
  Add/1 -> Max/2
  T/1 -> Relational Operator/1, Max/1
  Max/1 -> Unit Delay/1, Relational Operator/2
  Constant1/1 -> Discrete-Time Integrator1/1

== system Control_Logic_a/OST10 ==
  In : Inport  OutDataTypeStr=boolean  SampleTime=Sample_time
  T : Inport  Port=2  OutDataTypeStr=double  SampleTime=Sample_time
  Add : Sum  OutDataTypeStr=double
  Constant1 : Constant  SampleTime=Sample_time
  Discrete-Time Integrator1 : DiscreteIntegrator  SampleTime=Sample_time  LimitOutput=on  LowerSaturationLimit=0  ICPrevOutput=DiscIntNeverNeededParam  ICPrevScaledInput=DiscIntNeverNeededParam
  Logical Operator1 : Logic  AllPortsSameDT=off  OutDataTypeStr=boolean
  Max : MinMax  Inputs=2  OutDataTypeStr=double
  Parameter : Constant  Value=0  OutDataTypeStr=double  SampleTime=Sample_time
  Relational Operator : RelationalOperator  Operator=>  OutDataTypeStr=boolean  RndMeth=Nearest
  Sub : Sum  Inputs=+-  AccumDataTypeStr=single  OutDataTypeStr=double
  Switch : Switch  Criteria=u2 > Threshold  Threshold=0.5  OutDataTypeStr=double
  Unit Delay : UnitDelay  SampleTime=Sample_time
  Unit Delay2 : UnitDelay  InitialCondition=Ini_time  SampleTime=Sample_time
  Out : Outport  OutDataTypeStr=boolean  SampleTime=Sample_time
  wires:
  In/1 -> Switch/2, Logical Operator1/2
  Discrete-Time Integrator1/1 -> Unit Delay2/1, Sub/1
  Unit Delay2/1 -> Sub/2
  Sub/1 -> Add/1
  Logical Operator1/1 -> Out/1
  Relational Operator/1 -> Logical Operator1/1
  Switch/1 -> Add/2
  Unit Delay/1 -> Switch/1
  Parameter/1 -> Switch/3
  Add/1 -> Max/2
  T/1 -> Relational Operator/1, Max/1
  Max/1 -> Unit Delay/1, Relational Operator/2
  Constant1/1 -> Discrete-Time Integrator1/1

== system Control_Logic_a/OST11 ==
  In : Inport  OutDataTypeStr=boolean  SampleTime=Sample_time
  T : Inport  Port=2  OutDataTypeStr=double  SampleTime=Sample_time
  Add : Sum  OutDataTypeStr=double
  Constant1 : Constant  SampleTime=Sample_time
  Discrete-Time Integrator1 : DiscreteIntegrator  SampleTime=Sample_time  LimitOutput=on  LowerSaturationLimit=0  ICPrevOutput=DiscIntNeverNeededParam  ICPrevScaledInput=DiscIntNeverNeededParam
  Logical Operator1 : Logic  AllPortsSameDT=off  OutDataTypeStr=boolean
  Max : MinMax  Inputs=2  OutDataTypeStr=double
  Parameter : Constant  Value=0  OutDataTypeStr=double  SampleTime=Sample_time
  Relational Operator : RelationalOperator  Operator=>  OutDataTypeStr=boolean  RndMeth=Nearest
  Sub : Sum  Inputs=+-  AccumDataTypeStr=single  OutDataTypeStr=double
  Switch : Switch  Criteria=u2 > Threshold  Threshold=0.5  OutDataTypeStr=double
  Unit Delay : UnitDelay  SampleTime=Sample_time
  Unit Delay2 : UnitDelay  InitialCondition=Ini_time  SampleTime=Sample_time
  Out : Outport  OutDataTypeStr=boolean  SampleTime=Sample_time
  wires:
  Constant1/1 -> Discrete-Time Integrator1/1
  Max/1 -> Relational Operator/2, Unit Delay/1
  T/1 -> Max/1, Relational Operator/1
  Add/1 -> Max/2
  Parameter/1 -> Switch/3
  Unit Delay/1 -> Switch/1
  Switch/1 -> Add/2
  Relational Operator/1 -> Logical Operator1/1
  Logical Operator1/1 -> Out/1
  Sub/1 -> Add/1
  Unit Delay2/1 -> Sub/2
  Discrete-Time Integrator1/1 -> Sub/1, Unit Delay2/1
  In/1 -> Logical Operator1/2, Switch/2

== system Control_Logic_a/OST12 ==
  In : Inport  OutDataTypeStr=boolean  SampleTime=Sample_time
  T : Inport  Port=2  OutDataTypeStr=double  SampleTime=Sample_time
  Add : Sum  OutDataTypeStr=double
  Constant1 : Constant  SampleTime=Sample_time
  Discrete-Time Integrator1 : DiscreteIntegrator  SampleTime=Sample_time  LimitOutput=on  LowerSaturationLimit=0  ICPrevOutput=DiscIntNeverNeededParam  ICPrevScaledInput=DiscIntNeverNeededParam
  Logical Operator1 : Logic  AllPortsSameDT=off  OutDataTypeStr=boolean
  Max : MinMax  Inputs=2  OutDataTypeStr=double
  Parameter : Constant  Value=0  OutDataTypeStr=double  SampleTime=Sample_time
  Relational Operator : RelationalOperator  Operator=>  OutDataTypeStr=boolean  RndMeth=Nearest
  Sub : Sum  Inputs=+-  AccumDataTypeStr=single  OutDataTypeStr=double
  Switch : Switch  Criteria=u2 > Threshold  Threshold=0.5  OutDataTypeStr=double
  Unit Delay : UnitDelay  SampleTime=Sample_time
  Unit Delay2 : UnitDelay  InitialCondition=Ini_time  SampleTime=Sample_time
  Out : Outport  OutDataTypeStr=boolean  SampleTime=Sample_time
  wires:
  In/1 -> Switch/2, Logical Operator1/2
  Discrete-Time Integrator1/1 -> Unit Delay2/1, Sub/1
  Unit Delay2/1 -> Sub/2
  Sub/1 -> Add/1
  Logical Operator1/1 -> Out/1
  Relational Operator/1 -> Logical Operator1/1
  Switch/1 -> Add/2
  Unit Delay/1 -> Switch/1
  Parameter/1 -> Switch/3
  Add/1 -> Max/2
  T/1 -> Relational Operator/1, Max/1
  Max/1 -> Unit Delay/1, Relational Operator/2
  Constant1/1 -> Discrete-Time Integrator1/1

== system Control_Logic_a/OST13 ==
  In : Inport  OutDataTypeStr=boolean  SampleTime=Sample_time
  T : Inport  Port=2  OutDataTypeStr=double  SampleTime=Sample_time
  Add : Sum  OutDataTypeStr=double
  Constant1 : Constant  SampleTime=Sample_time
  Discrete-Time Integrator1 : DiscreteIntegrator  SampleTime=Sample_time  LimitOutput=on  LowerSaturationLimit=0  ICPrevOutput=DiscIntNeverNeededParam  ICPrevScaledInput=DiscIntNeverNeededParam
  Logical Operator1 : Logic  AllPortsSameDT=off  OutDataTypeStr=boolean
  Max : MinMax  Inputs=2  OutDataTypeStr=double
  Parameter : Constant  Value=0  OutDataTypeStr=double  SampleTime=Sample_time
  Relational Operator : RelationalOperator  Operator=>  OutDataTypeStr=boolean  RndMeth=Nearest
  Sub : Sum  Inputs=+-  AccumDataTypeStr=single  OutDataTypeStr=double
  Switch : Switch  Criteria=u2 > Threshold  Threshold=0.5  OutDataTypeStr=double
  Unit Delay : UnitDelay  SampleTime=Sample_time
  Unit Delay2 : UnitDelay  InitialCondition=Ini_time  SampleTime=Sample_time
  Out : Outport  OutDataTypeStr=boolean  SampleTime=Sample_time
  wires:
  Constant1/1 -> Discrete-Time Integrator1/1
  Max/1 -> Relational Operator/2, Unit Delay/1
  T/1 -> Max/1, Relational Operator/1
  Add/1 -> Max/2
  Parameter/1 -> Switch/3
  Unit Delay/1 -> Switch/1
  Switch/1 -> Add/2
  Relational Operator/1 -> Logical Operator1/1
  Logical Operator1/1 -> Out/1
  Sub/1 -> Add/1
  Unit Delay2/1 -> Sub/2
  Discrete-Time Integrator1/1 -> Sub/1, Unit Delay2/1
  In/1 -> Logical Operator1/2, Switch/2

== system Control_Logic_a/OST14 ==
  In : Inport  OutDataTypeStr=boolean  SampleTime=Sample_time
  T : Inport  Port=2  OutDataTypeStr=double  SampleTime=Sample_time
  Add : Sum  OutDataTypeStr=double
  Constant1 : Constant  SampleTime=Sample_time
  Discrete-Time Integrator1 : DiscreteIntegrator  SampleTime=Sample_time  LimitOutput=on  LowerSaturationLimit=0  ICPrevOutput=DiscIntNeverNeededParam  ICPrevScaledInput=DiscIntNeverNeededParam
  Logical Operator1 : Logic  AllPortsSameDT=off  OutDataTypeStr=boolean
  Max : MinMax  Inputs=2  OutDataTypeStr=double
  Parameter : Constant  Value=0  OutDataTypeStr=double  SampleTime=Sample_time
  Relational Operator : RelationalOperator  Operator=>  OutDataTypeStr=boolean  RndMeth=Nearest
  Sub : Sum  Inputs=+-  AccumDataTypeStr=single  OutDataTypeStr=double
  Switch : Switch  Criteria=u2 > Threshold  Threshold=0.5  OutDataTypeStr=double
  Unit Delay : UnitDelay  SampleTime=Sample_time
  Unit Delay2 : UnitDelay  InitialCondition=Ini_time  SampleTime=Sample_time
  Out : Outport  OutDataTypeStr=boolean  SampleTime=Sample_time
  wires:
  Max/1 -> Relational Operator/2, Unit Delay/1
  T/1 -> Max/1, Relational Operator/1
  Add/1 -> Max/2
  Parameter/1 -> Switch/3
  Unit Delay/1 -> Switch/1
  Switch/1 -> Add/2
  Relational Operator/1 -> Logical Operator1/1
  Logical Operator1/1 -> Out/1
  Sub/1 -> Add/1
  Unit Delay2/1 -> Sub/2
  Discrete-Time Integrator1/1 -> Sub/1, Unit Delay2/1
  In/1 -> Logical Operator1/2, Switch/2
  Constant1/1 -> Discrete-Time Integrator1/1

== system Control_Logic_a/OST15 ==
  In : Inport  OutDataTypeStr=boolean  SampleTime=Sample_time
  T : Inport  Port=2  OutDataTypeStr=double  SampleTime=Sample_time
  Add : Sum  OutDataTypeStr=double
  Constant1 : Constant  SampleTime=Sample_time
  Discrete-Time Integrator1 : DiscreteIntegrator  SampleTime=Sample_time  LimitOutput=on  LowerSaturationLimit=0  ICPrevOutput=DiscIntNeverNeededParam  ICPrevScaledInput=DiscIntNeverNeededParam
  Logical Operator1 : Logic  AllPortsSameDT=off  OutDataTypeStr=boolean
  Max : MinMax  Inputs=2  OutDataTypeStr=double
  Parameter : Constant  Value=0  OutDataTypeStr=double  SampleTime=Sample_time
  Relational Operator : RelationalOperator  Operator=>  OutDataTypeStr=boolean  RndMeth=Nearest
  Sub : Sum  Inputs=+-  AccumDataTypeStr=single  OutDataTypeStr=double
  Switch : Switch  Criteria=u2 > Threshold  Threshold=0.5  OutDataTypeStr=double
  Unit Delay : UnitDelay  SampleTime=Sample_time
  Unit Delay2 : UnitDelay  InitialCondition=Ini_time  SampleTime=Sample_time
  Out : Outport  OutDataTypeStr=boolean  SampleTime=Sample_time
  wires:
  Constant1/1 -> Discrete-Time Integrator1/1
  In/1 -> Switch/2, Logical Operator1/2
  Discrete-Time Integrator1/1 -> Unit Delay2/1, Sub/1
  Unit Delay2/1 -> Sub/2
  Sub/1 -> Add/1
  Logical Operator1/1 -> Out/1
  Relational Operator/1 -> Logical Operator1/1
  Switch/1 -> Add/2
  Unit Delay/1 -> Switch/1
  Parameter/1 -> Switch/3
  Add/1 -> Max/2
  T/1 -> Relational Operator/1, Max/1
  Max/1 -> Unit Delay/1, Relational Operator/2

== system Control_Logic_a/OST16 ==
  In : Inport  OutDataTypeStr=boolean  SampleTime=Sample_time
  T : Inport  Port=2  OutDataTypeStr=double  SampleTime=Sample_time
  Add : Sum  OutDataTypeStr=double
  Constant1 : Constant  SampleTime=Sample_time
  Discrete-Time Integrator1 : DiscreteIntegrator  SampleTime=Sample_time  LimitOutput=on  LowerSaturationLimit=0  ICPrevOutput=DiscIntNeverNeededParam  ICPrevScaledInput=DiscIntNeverNeededParam
  Logical Operator1 : Logic  AllPortsSameDT=off  OutDataTypeStr=boolean
  Max : MinMax  Inputs=2  OutDataTypeStr=double
  Parameter : Constant  Value=0  OutDataTypeStr=double  SampleTime=Sample_time
  Relational Operator : RelationalOperator  Operator=>  OutDataTypeStr=boolean  RndMeth=Nearest
  Sub : Sum  Inputs=+-  AccumDataTypeStr=single  OutDataTypeStr=double
  Switch : Switch  Criteria=u2 > Threshold  Threshold=0.5  OutDataTypeStr=double
  Unit Delay : UnitDelay  SampleTime=Sample_time
  Unit Delay2 : UnitDelay  InitialCondition=Ini_time  SampleTime=Sample_time
  Out : Outport  OutDataTypeStr=boolean  SampleTime=Sample_time
  wires:
  Max/1 -> Relational Operator/2, Unit Delay/1
  T/1 -> Max/1, Relational Operator/1
  Add/1 -> Max/2
  Parameter/1 -> Switch/3
  Unit Delay/1 -> Switch/1
  Switch/1 -> Add/2
  Relational Operator/1 -> Logical Operator1/1
  Logical Operator1/1 -> Out/1
  Sub/1 -> Add/1
  Unit Delay2/1 -> Sub/2
  Discrete-Time Integrator1/1 -> Sub/1, Unit Delay2/1
  In/1 -> Logical Operator1/2, Switch/2
  Constant1/1 -> Discrete-Time Integrator1/1

== system Control_Logic_a/OST2 ==
  In : Inport  OutDataTypeStr=boolean  SampleTime=Sample_time
  T : Inport  Port=2  OutDataTypeStr=double  SampleTime=Sample_time
  Add : Sum  OutDataTypeStr=double
  Constant1 : Constant  SampleTime=Sample_time
  Discrete-Time Integrator1 : DiscreteIntegrator  SampleTime=Sample_time  LimitOutput=on  LowerSaturationLimit=0  ICPrevOutput=DiscIntNeverNeededParam  ICPrevScaledInput=DiscIntNeverNeededParam
  Logical Operator1 : Logic  AllPortsSameDT=off  OutDataTypeStr=boolean
  Max : MinMax  Inputs=2  OutDataTypeStr=double
  Parameter : Constant  Value=0  OutDataTypeStr=double  SampleTime=Sample_time
  Relational Operator : RelationalOperator  Operator=>  OutDataTypeStr=boolean  RndMeth=Nearest
  Sub : Sum  Inputs=+-  AccumDataTypeStr=single  OutDataTypeStr=double
  Switch : Switch  Criteria=u2 > Threshold  Threshold=0.5  OutDataTypeStr=double
  Unit Delay : UnitDelay  SampleTime=Sample_time
  Unit Delay2 : UnitDelay  InitialCondition=Ini_time  SampleTime=Sample_time
  Out : Outport  OutDataTypeStr=boolean  SampleTime=Sample_time
  wires:
  Max/1 -> Relational Operator/2, Unit Delay/1
  T/1 -> Max/1, Relational Operator/1
  Add/1 -> Max/2
  Parameter/1 -> Switch/3
  Unit Delay/1 -> Switch/1
  Switch/1 -> Add/2
  Relational Operator/1 -> Logical Operator1/1
  Logical Operator1/1 -> Out/1
  Sub/1 -> Add/1
  Unit Delay2/1 -> Sub/2
  Discrete-Time Integrator1/1 -> Sub/1, Unit Delay2/1
  In/1 -> Logical Operator1/2, Switch/2
  Constant1/1 -> Discrete-Time Integrator1/1

== system Control_Logic_a/OST3 ==
  In : Inport  OutDataTypeStr=boolean  SampleTime=Sample_time
  T : Inport  Port=2  OutDataTypeStr=double  SampleTime=Sample_time
  Add : Sum  OutDataTypeStr=double
  Constant1 : Constant  SampleTime=Sample_time
  Discrete-Time Integrator1 : DiscreteIntegrator  SampleTime=Sample_time  LimitOutput=on  LowerSaturationLimit=0  ICPrevOutput=DiscIntNeverNeededParam  ICPrevScaledInput=DiscIntNeverNeededParam
  Logical Operator1 : Logic  AllPortsSameDT=off  OutDataTypeStr=boolean
  Max : MinMax  Inputs=2  OutDataTypeStr=double
  Parameter : Constant  Value=0  OutDataTypeStr=double  SampleTime=Sample_time
  Relational Operator : RelationalOperator  Operator=>  OutDataTypeStr=boolean  RndMeth=Nearest
  Sub : Sum  Inputs=+-  AccumDataTypeStr=single  OutDataTypeStr=double
  Switch : Switch  Criteria=u2 > Threshold  Threshold=0.5  OutDataTypeStr=double
  Unit Delay : UnitDelay  SampleTime=Sample_time
  Unit Delay2 : UnitDelay  InitialCondition=Ini_time  SampleTime=Sample_time
  Out : Outport  OutDataTypeStr=boolean  SampleTime=Sample_time
  wires:
  Max/1 -> Relational Operator/2, Unit Delay/1
  T/1 -> Max/1, Relational Operator/1
  Add/1 -> Max/2
  Parameter/1 -> Switch/3
  Unit Delay/1 -> Switch/1
  Switch/1 -> Add/2
  Relational Operator/1 -> Logical Operator1/1
  Logical Operator1/1 -> Out/1
  Sub/1 -> Add/1
  Unit Delay2/1 -> Sub/2
  Discrete-Time Integrator1/1 -> Sub/1, Unit Delay2/1
  In/1 -> Logical Operator1/2, Switch/2
  Constant1/1 -> Discrete-Time Integrator1/1

== system Control_Logic_a/OST4 ==
  In : Inport  OutDataTypeStr=boolean  SampleTime=Sample_time
  T : Inport  Port=2  OutDataTypeStr=double  SampleTime=Sample_time
  Add : Sum  OutDataTypeStr=double
  Constant1 : Constant  SampleTime=Sample_time
  Discrete-Time Integrator1 : DiscreteIntegrator  SampleTime=Sample_time  LimitOutput=on  LowerSaturationLimit=0  ICPrevOutput=DiscIntNeverNeededParam  ICPrevScaledInput=DiscIntNeverNeededParam
  Logical Operator1 : Logic  AllPortsSameDT=off  OutDataTypeStr=boolean
  Max : MinMax  Inputs=2  OutDataTypeStr=double
  Parameter : Constant  Value=0  OutDataTypeStr=double  SampleTime=Sample_time
  Relational Operator : RelationalOperator  Operator=>  OutDataTypeStr=boolean  RndMeth=Nearest
  Sub : Sum  Inputs=+-  AccumDataTypeStr=single  OutDataTypeStr=double
  Switch : Switch  Criteria=u2 > Threshold  Threshold=0.5  OutDataTypeStr=double
  Unit Delay : UnitDelay  SampleTime=Sample_time
  Unit Delay2 : UnitDelay  InitialCondition=Ini_time  SampleTime=Sample_time
  Out : Outport  OutDataTypeStr=boolean  SampleTime=Sample_time
  wires:
  In/1 -> Switch/2, Logical Operator1/2
  Discrete-Time Integrator1/1 -> Unit Delay2/1, Sub/1
  Unit Delay2/1 -> Sub/2
  Sub/1 -> Add/1
  Logical Operator1/1 -> Out/1
  Relational Operator/1 -> Logical Operator1/1
  Switch/1 -> Add/2
  Unit Delay/1 -> Switch/1
  Parameter/1 -> Switch/3
  Add/1 -> Max/2
  T/1 -> Relational Operator/1, Max/1
  Max/1 -> Unit Delay/1, Relational Operator/2
  Constant1/1 -> Discrete-Time Integrator1/1

== system Control_Logic_a/OST5 ==
  In : Inport  OutDataTypeStr=boolean  SampleTime=Sample_time
  T : Inport  Port=2  OutDataTypeStr=double  SampleTime=Sample_time
  Add : Sum  OutDataTypeStr=double
  Constant1 : Constant  SampleTime=Sample_time
  Discrete-Time Integrator1 : DiscreteIntegrator  SampleTime=Sample_time  LimitOutput=on  LowerSaturationLimit=0  ICPrevOutput=DiscIntNeverNeededParam  ICPrevScaledInput=DiscIntNeverNeededParam
  Logical Operator1 : Logic  AllPortsSameDT=off  OutDataTypeStr=boolean
  Max : MinMax  Inputs=2  OutDataTypeStr=double
  Parameter : Constant  Value=0  OutDataTypeStr=double  SampleTime=Sample_time
  Relational Operator : RelationalOperator  Operator=>  OutDataTypeStr=boolean  RndMeth=Nearest
  Sub : Sum  Inputs=+-  AccumDataTypeStr=single  OutDataTypeStr=double
  Switch : Switch  Criteria=u2 > Threshold  Threshold=0.5  OutDataTypeStr=double
  Unit Delay : UnitDelay  SampleTime=Sample_time
  Unit Delay2 : UnitDelay  InitialCondition=Ini_time  SampleTime=Sample_time
  Out : Outport  OutDataTypeStr=boolean  SampleTime=Sample_time
  wires:
  Max/1 -> Relational Operator/2, Unit Delay/1
  T/1 -> Max/1, Relational Operator/1
  Add/1 -> Max/2
  Parameter/1 -> Switch/3
  Unit Delay/1 -> Switch/1
  Switch/1 -> Add/2
  Relational Operator/1 -> Logical Operator1/1
  Logical Operator1/1 -> Out/1
  Sub/1 -> Add/1
  Unit Delay2/1 -> Sub/2
  Discrete-Time Integrator1/1 -> Sub/1, Unit Delay2/1
  In/1 -> Logical Operator1/2, Switch/2
  Constant1/1 -> Discrete-Time Integrator1/1

== system Control_Logic_a/OST6 ==
  In : Inport  OutDataTypeStr=boolean  SampleTime=Sample_time
  T : Inport  Port=2  OutDataTypeStr=double  SampleTime=Sample_time
  Add : Sum  OutDataTypeStr=double
  Constant1 : Constant  SampleTime=Sample_time
  Discrete-Time Integrator1 : DiscreteIntegrator  SampleTime=Sample_time  LimitOutput=on  LowerSaturationLimit=0  ICPrevOutput=DiscIntNeverNeededParam  ICPrevScaledInput=DiscIntNeverNeededParam
  Logical Operator1 : Logic  AllPortsSameDT=off  OutDataTypeStr=boolean
  Max : MinMax  Inputs=2  OutDataTypeStr=double
  Parameter : Constant  Value=0  OutDataTypeStr=double  SampleTime=Sample_time
  Relational Operator : RelationalOperator  Operator=>  OutDataTypeStr=boolean  RndMeth=Nearest
  Sub : Sum  Inputs=+-  AccumDataTypeStr=single  OutDataTypeStr=double
  Switch : Switch  Criteria=u2 > Threshold  Threshold=0.5  OutDataTypeStr=double
  Unit Delay : UnitDelay  SampleTime=Sample_time
  Unit Delay2 : UnitDelay  InitialCondition=Ini_time  SampleTime=Sample_time
  Out : Outport  OutDataTypeStr=boolean  SampleTime=Sample_time
  wires:
  In/1 -> Switch/2, Logical Operator1/2
  Discrete-Time Integrator1/1 -> Unit Delay2/1, Sub/1
  Unit Delay2/1 -> Sub/2
  Sub/1 -> Add/1
  Logical Operator1/1 -> Out/1
  Relational Operator/1 -> Logical Operator1/1
  Switch/1 -> Add/2
  Unit Delay/1 -> Switch/1
  Parameter/1 -> Switch/3
  Add/1 -> Max/2
  T/1 -> Relational Operator/1, Max/1
  Max/1 -> Unit Delay/1, Relational Operator/2
  Constant1/1 -> Discrete-Time Integrator1/1
